simulink model "pva1"  (R2019b)
settings: Solver=FixedStepAuto  StartTime=0.0  StopTime=30  FixedStep=0.01  RelTol=1e-3
settings Model: Creator=suvo  LastModifiedBy=suvo

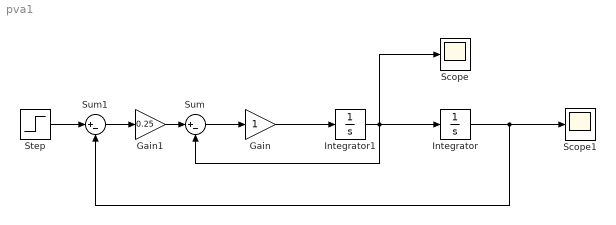
== system pva1 ==
  Gain : Gain
  Gain1 : Gain  Gain=0.25
  Integrator : Integrator
  Integrator1 : Integrator
  Scope : Scope
  Scope1 : Scope
  Step : Step  SampleTime=0
  Sum : Sum  Inputs=|+-
  Sum1 : Sum  Inputs=|+-
  wires:
  Sum/1 -> Gain/1
  Gain/1 -> Integrator1/1
  Integrator1/1 -> Integrator/1, Sum/2, Scope/1
  Gain1/1 -> Sum/1
  Sum1/1 -> Gain1/1
  Step/1 -> Sum1/1
  Integrator/1 -> Scope1/1, Sum1/2
